simulink model "car_control_byJoystick"  (R2023a)
settings: Solver=VariableStepAuto  StartTime=0.0  StopTime=10.0  RelTol=1e-3
libraries: vrlib x1
settings Model: Creator=15113  LastModifiedBy=15113

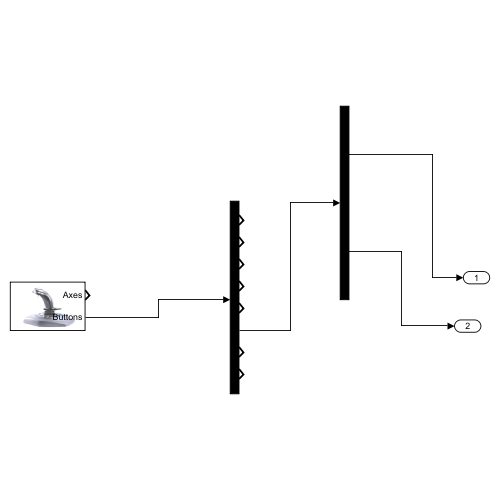
[thumbnail: Simulink's stored preview of the top-level diagram]
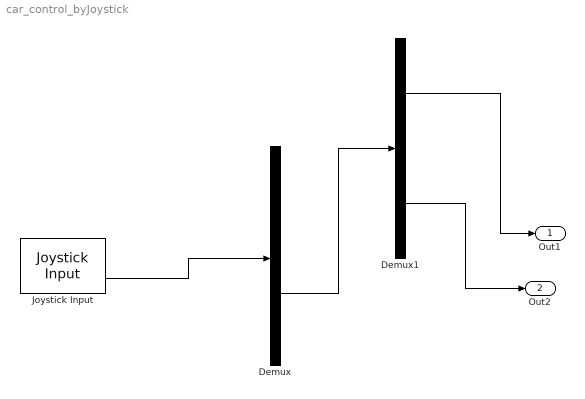
== system car_control_byJoystick ==
  Demux : Demux  Outputs=8
  Demux1 : Demux  Outputs=2
  Joystick Input : vrlib/Joystick Input  joyid=1  adjustports=on  forcefeed=off
  Out1 : Outport
  Out2 : Outport  Port=2
  wires:
  Demux1/1 -> Out1/1
  Demux/6 -> Demux1/1
  Demux1/2 -> Out2/1
  Joystick Input/2 -> Demux/1
